simulink model "NDM"  (Simulink 7.7)
settings: Solver=ode3  StartTime=0.0  StopTime=100000  FixedStep=0.1  RelTol=1e-3
settings Model: Creator=PC  LastModifiedBy=Natalia
settings OptimizationCC: ExpressionDepthLimit=128
settings DebuggingCC: MultiTaskDSMMsg=warning  MultiTaskCondExecSysMsg=none  StrictBusMsg=None
settings RTWCC: IncludeERTFirstTime=on
settings CodeAppCC: CustomSymbolStrType=$N$R$M_T
settings GRTTargetCC: CombineOutputUpdateFcns=on  CPPClassGenCompliant=on

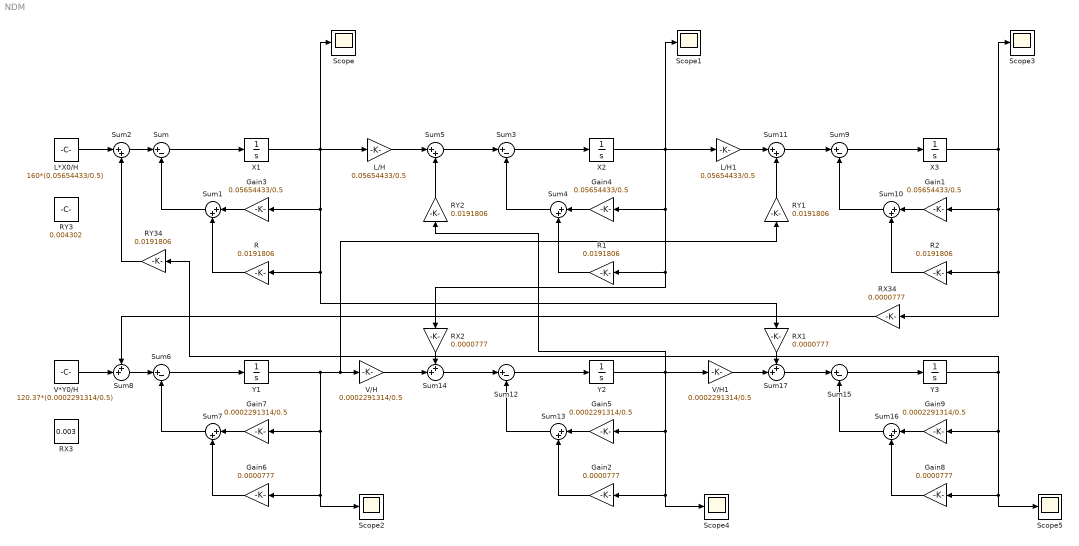
== system NDM ==
  Gain1 : Gain  Gain=0.05654433/0.5
  Gain2 : Gain  Gain=0.0000777
  Gain3 : Gain  Gain=0.05654433/0.5
  Gain4 : Gain  Gain=0.05654433/0.5
  Gain5 : Gain  Gain=0.0002291314/0.5
  Gain6 : Gain  Gain=0.0000777
  Gain7 : Gain  Gain=0.0002291314/0.5
  Gain8 : Gain  Gain=0.0000777
  Gain9 : Gain  Gain=0.0002291314/0.5
  L*X0/H : Constant  Value=160*(0.05654433/0.5)
  L/H : Gain  Gain=0.05654433/0.5
  L/H1 : Gain  Gain=0.05654433/0.5
  R : Gain  Gain=0.0191806
  R1 : Gain  Gain=0.0191806
  R2 : Gain  Gain=0.0191806
  RX1 : Gain  Gain=0.0000777
  RX2 : Gain  Gain=0.0000777
  RX3 : Constant  Value=0.003
  RX34 : Gain  Gain=0.0000777
  RY1 : Gain  Gain=0.0191806
  RY2 : Gain  Gain=0.0191806
  RY3 : Constant  Value=0.004302
  RY34 : Gain  Gain=0.0191806
  Scope{,1..5} (6 alike) : Scope
      Scope settings: YMin=152  YMax=168
      Scope1 settings: YMin=152  YMax=168
      Scope2 settings: YMin=-0.00145  YMax=-0.0003  SaveName=ScopeData2
      Scope3 settings: SaveName=ScopeData3
      Scope4 settings: YMin=-0.0196  YMax=-0.0181  SaveName=ScopeData4
      Scope5 settings: SaveName=ScopeData5
  Sum{,3,6,9,12,15} (6 alike) : Sum  Inputs=|+-
  Sum{1..2,4..5,7,10..11,13,16} (9 alike) : Sum  Inputs=|++
  Sum14 : Sum  Inputs=++|
  Sum17 : Sum  Inputs=++|
  Sum8 : Sum  Inputs=++|
  V*Y0/H : Constant  Value=120.37*(0.0002291314/0.5)
  V/H : Gain  Gain=0.0002291314/0.5
  V/H1 : Gain  Gain=0.0002291314/0.5
  X1 : Integrator
  X2 : Integrator
  X3 : Integrator
  Y1 : Integrator
  Y2 : Integrator
  Y3 : Integrator
  wires:
  Gain3/1 -> Sum1/1
  R/1 -> Sum1/2
  Sum/1 -> X1/1
  X1/1 -> L/H/1, Scope/1, RX1/1, R/1, Gain3/1
  Sum1/1 -> Sum/2
  Sum2/1 -> Sum/1
  L*X0/H/1 -> Sum2/1
  Gain4/1 -> Sum4/1
  R1/1 -> Sum4/2
  Sum3/1 -> X2/1
  X2/1 -> L/H1/1, Scope1/1, RX2/1, R1/1, Gain4/1
  Sum4/1 -> Sum3/2
  Sum5/1 -> Sum3/1
  L/H/1 -> Sum5/1
  Gain7/1 -> Sum7/1
  Gain6/1 -> Sum7/2
  Sum6/1 -> Y1/1
  Y1/1 -> RY1/1, V/H/1, Scope2/1, Gain6/1, Gain7/1
  Sum7/1 -> Sum6/2
  Sum8/1 -> Sum6/1
  Gain1/1 -> Sum10/1
  R2/1 -> Sum10/2
  Sum9/1 -> X3/1
  X3/1 -> Scope3/1, RX34/1, R2/1, Gain1/1
  Sum10/1 -> Sum9/2
  RY1/1 -> Sum11/2
  Sum11/1 -> Sum9/1
  L/H1/1 -> Sum11/1
  Gain5/1 -> Sum13/1
  Gain2/1 -> Sum13/2
  Sum12/1 -> Y2/1
  Y2/1 -> Scope4/1, Gain2/1, Gain5/1, V/H1/1, RY2/1
  Sum13/1 -> Sum12/2
  Sum14/1 -> Sum12/1
  Gain9/1 -> Sum16/1
  Gain8/1 -> Sum16/2
  Sum15/1 -> Y3/1
  Sum16/1 -> Sum15/2
  Sum17/1 -> Sum15/1
  RY2/1 -> Sum5/2
  V/H/1 -> Sum14/2
  RX2/1 -> Sum14/1
  V/H1/1 -> Sum17/2
  RX1/1 -> Sum17/1
  RY34/1 -> Sum2/2
  Y3/1 -> RY34/1, Scope5/1, Gain8/1, Gain9/1
  RX34/1 -> Sum8/1
  V*Y0/H/1 -> Sum8/2
